simulink model "simulacao_pid_compatibilidade"  (Simulink 7.7)
settings: Solver=ode4  SolverMode=SingleTasking  StartTime=0.0  StopTime=100.0  FixedStep=0.002  RelTol=1e-3
libraries: simulink x3
settings Model: Creator=root  LastModifiedBy=root  CovMetricSettings=dwe  CovHtmlReporting=off  covSaveCumulativeToWorkspaceVar=off  CovSaveSingleToWorkspaceVar=off  CovExternalEMLEnable=on
settings DataIOCC: LimitDataPoints=off  SaveFormat=StructureWithTime  SignalLoggingSaveFormat=Dataset
settings OptimizationCC: ExpressionDepthLimit=128
settings DebuggingCC: UnderspecifiedInitializationDetection=Simplified  MergeDetectMultiDrivingBlocksExec=error  SolverPrmCheckMsg=none  FcnCallInpInsideContextMsg=Enable All  StateNameClashWarn=none  SFUnexpectedBacktrackingDiag=error  SFNoUnconditionalDefaultTransitionDiag=error
settings HardwareCC: ProdBitPerPointer=64  ProdLargestAtomicFloat=Float  ProdIntDivRoundTo=Zero  ProdEndianess=LittleEndian  ProdHWDeviceType=Specified
settings CodeAppCC: CustomSymbolStrType=$N$R$M_T
settings GRTTargetCC: TargetFunctionLibrary=C99 (ISO)  GeneratePreprocessorConditionals=Use local settings

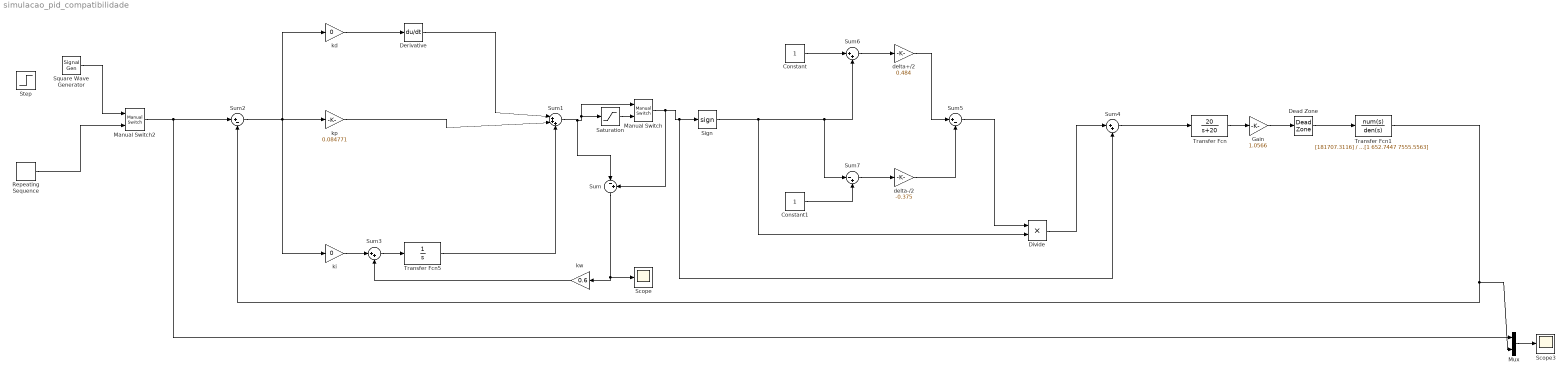
== system simulacao_pid_compatibilidade ==
  Constant : Constant
  Constant1 : Constant
  Dead Zone : DeadZone  LowerValue=-0.75  UpperValue=0.968  SaturateOnIntegerOverflow=on
  Derivative : Derivative
  Divide : Product  Inputs=**
  Gain : Gain  Gain=1.0566
  Manual Switch : simulink/Signal Routing/Manual Switch  sw=0  action=0  varsize=off
  Manual Switch2 : simulink/Signal Routing/Manual Switch  sw=1  action=0  varsize=off
  Mux : Mux  Inputs=2
  Repeating Sequence : simulink/Sources/Repeating Sequence  rep_seq_t=[0 2 4 96 98 100]  rep_seq_y=[0 1 0 0 -1 0]
  Saturation : Saturate  UpperLimit=10  LowerLimit=-10
  Scope : Scope
      settings: TimeRange=auto  MaxDataPoints=5000  SaveToWorkspace=off  YMin=-1275.63078  YMax=1275.62457  SampleTime=-1
  Scope3 : Scope
      settings: TimeRange=auto  MaxDataPoints=5000  SaveToWorkspace=off  SaveName=ScopeData3  YMin=-66.39975  YMax=66.39975  SampleTime=-1
  Sign : Signum
  Square Wave Generator : SignalGenerator  WaveForm=square  Amplitude=45  Units=rad/sec
  Step : Step  After=10  SampleTime=0
  Sum : Sum  Inputs=|-+
  Sum1 : Sum  Inputs=|+++
  Sum2 : Sum  Inputs=|+-
  Sum3 : Sum  Inputs=|++
  Sum4 : Sum  Inputs=|++
  Sum5 : Sum  Inputs=|+-
  Sum6 : Sum  Inputs=|++
  Sum7 : Sum  Inputs=|-+
  Transfer Fcn : TransferFcn  Numerator=[20]  Denominator=[1 20]
  Transfer Fcn1 : TransferFcn  Numerator=[181707.3116]  Denominator=[1 652.7447 7555.5563]
  Transfer Fcn5 : TransferFcn  Denominator=[1 0]
  delta+/2 : Gain  Gain=0.484
  delta-/2 : Gain  Gain=-0.375
  "kd " : Gain  Gain=0
  ki : Gain  Gain=0
  kp : Gain  Gain=0.084771
  kw : Gain  Gain=0.6
  wires:
  Transfer Fcn/1 -> Gain/1
  Dead Zone/1 -> Transfer Fcn1/1
  Mux/1 -> Scope3/1
  Gain/1 -> Dead Zone/1
  Repeating Sequence/1 -> Manual Switch2/2
  Manual Switch2/1 -> Mux/1, Sum2/1
  Sum2/1 -> "kd "/1, ki/1, kp/1
  kp/1 -> Sum1/2
  "kd "/1 -> Derivative/1
  Derivative/1 -> Sum1/1
  Transfer Fcn5/1 -> Sum1/3
  Sum1/1 -> Manual Switch/1, Saturation/1, Sum/1
  ki/1 -> Sum3/1
  Sum3/1 -> Transfer Fcn5/1
  Sign/1 -> Divide/2, Sum7/1, Sum6/2
  Sum6/1 -> delta+/2/1
  Sum7/1 -> delta-/2/1
  delta-/2/1 -> Sum5/2
  delta+/2/1 -> Sum5/1
  Sum5/1 -> Divide/1
  Divide/1 -> Sum4/1
  Constant1/1 -> Sum7/2
  Constant/1 -> Sum6/1
  Sum4/1 -> Transfer Fcn/1
  Sum/1 -> Scope/1, kw/1
  kw/1 -> Sum3/2
  Square Wave Generator/1 -> Manual Switch2/1
  Saturation/1 -> Manual Switch/2
  Manual Switch/1 -> Sum/2, Sum4/2, Sign/1
  Transfer Fcn1/1 -> Mux/2, Sum2/2
